simulink model "run_sim_paper_scenario"  (R2020a)
settings: Solver=ode4  StartTime=0.0  StopTime=30.0  FixedStep=0.01  RelTol=1e-3
values from neighbouring files (symbols this model uses):
  alfa_theta = 20    [init_sim_paper_scenario.m]
  alfa_theta_obs = 100    [init_sim_paper_scenario.m]
  beta1 = 1.2    [init_sim_paper_scenario.m]
  beta2 = 0.8    [init_sim_paper_scenario.m]
  beta_Phi_1 = pp0 * cal_frac_squ( 3, p_p0_plus_1, q_p0_plus_1 )                          * cal_frac_squ( eps_s_bar / pi, p_p0_min_2, q_p0_min_2 )                          / ( 2 * ( 2 * pp0 - 1 ) * tanh( gamma0 * ( eps_s_bar / pi ) / 2 ) )                          - ( cal_frac_squ( 3, p_p0_plus_1, q_p0_plus_1 ) * gamma0 / ( 4 * ( 2 * pp0 -1 ) ) )                          * cal_frac_squ( eps_s_bar / pi, p_p0_min_ ...(+136 chars)    [init_sim_paper_scenario.m]
  beta_Phi_2 = ( 1 - pp0 ) * cal_frac_squ( 3, p_p0_plus_1, q_p0_plus_1 )                          / ( 2 * ( 1 - 2 * pp0 ) * cal_frac_squ( eps_s_bar / pi, p_p0_0, q_p0_0 ) * tanh( gamma0 * ( eps_s_bar / pi ) / 2 ) )                          - ( cal_frac_squ( 3, p_p0_plus_1, q_p0_plus_1 ) * gamma0 / ( 4 * ( 1 - 2 * pp0 ) ) )                          * cal_frac_squ( eps_s_bar / pi, p_1_min_p0, q_1_min_p0 )          ...(+112 chars)    [init_sim_paper_scenario.m]
  c1_diff_sigma_bar_v = diag([25; 30; 20])    [init_sim_paper_scenario.m]
  c1_diff_sigma_bar_w = diag([12; 12; 12])    [init_sim_paper_scenario.m]
  c1_diff_ui = diag([25; 30; 20])    [init_sim_paper_scenario.m]
  c1v = diag([5.8; 6.5; 6.5])    [init_sim_paper_scenario.m]
  c2_diff_sigma_bar_v = diag([50; 50; 10])    [init_sim_paper_scenario.m]
  c2_diff_sigma_bar_w = diag([12; 12; 12])    [init_sim_paper_scenario.m]
  c2_diff_ui = diag([50; 50; 10])    [init_sim_paper_scenario.m]
  c2v = diag([5.8; 6.5; 6.5])    [init_sim_paper_scenario.m]
  c3_diff_sigma_bar_v = diag([15; 15; 10])    [init_sim_paper_scenario.m]
  c3_diff_sigma_bar_w = diag([15; 15; 15])    [init_sim_paper_scenario.m]
  c3_diff_ui = diag([15; 15; 10])    [init_sim_paper_scenario.m]
  c3v = diag([4.8; 6.4; 6.0])    [init_sim_paper_scenario.m]
  c_w_1 = diag( [20; 15; 15] )    [init_sim_paper_scenario.m]
  c_w_2 = diag( [20; 15; 15] )    [init_sim_paper_scenario.m]
  c_w_3 = diag( [2; 2; 2] )    [init_sim_paper_scenario.m]
  cS0 = diag( [4.5; 4.5; 4.5] )    [init_sim_paper_scenario.m]
  delta_p_i_0 = zeros(3, NF)    [init_sim_paper_scenario.m]
  delta_v_i_0 = zeros(3, NF)    [init_sim_paper_scenario.m]
  dp_aa_t = 0.2 * ones(3, 5) + ( 1.0 - 0.2 ) * rand(3, 5)    [init_sim_paper_scenario.m]
  dp_ff_t = [ 0.4 * ones(1, 5) + ( 1.0 - 0.4 ) * rand(1, 5);                      0.4 * ones(1, 5) + ( 1.0 - 0.4 ) * rand(1, 5);                      0.2 * ones(1, 5) + ( 0.6 - 0.2 ) * rand(1, 5) ]    [init_sim_paper_scenario.m]
  dp_phi_t = ( - pi / 2 ) * ones(3, 5) + ( pi / 2 - ( - pi / 2 ) ) * rand(3, 5)    [init_sim_paper_scenario.m]
  dw_aa_t = 0.2 * ones(3, 5) + ( 1.0 - 0.2 ) * rand(3, 5)    [init_sim_paper_scenario.m]
  dw_ff_t = [ 0.4 * ones(1, 5) + ( 1.0 - 0.4 ) * rand(1, 5);                      0.4 * ones(1, 5) + ( 1.0 - 0.4 ) * rand(1, 5);                      0.2 * ones(1, 5) + ( 0.6 - 0.2 ) * rand(1, 5) ]    [init_sim_paper_scenario.m]
  dw_phi_t = ( - pi / 2 ) * ones(3, 5) + ( pi / 2 - ( - pi / 2 ) ) * rand(3, 5)    [init_sim_paper_scenario.m]
  dwci_init = zeros(3,5)    [init_sim_paper_scenario.m]
  eps_s_bar_div_pi = eps_s_bar / pi    (= 0.03)    [init_sim_paper_scenario.m]
  etai_0 = zeros(3,5)    [init_sim_paper_scenario.m]
  gamma0 = 20    [init_sim_paper_scenario.m]
  h1w = diag([20.0; 20.0; 20.0])    [init_sim_paper_scenario.m]
  h2w = diag([30.0; 35.0; 35.0])    [init_sim_paper_scenario.m]
  h3w = diag([30.0; 25.0; 30.0])    [init_sim_paper_scenario.m]
  Ji = zeros(3,3,NF)    [init_sim_paper_scenario.m]
  k_J_0 = diag( [1; 1; 1] )    [init_sim_paper_scenario.m]
  kai_1_t = 0.02    [init_sim_paper_scenario.m]
  kai_3_t = 0.1    [init_sim_paper_scenario.m]
  kai_chi_1 = diag([6; 6; 6])    [init_sim_paper_scenario.m]
  kai_chi_2 = diag([6; 6; 6])    [init_sim_paper_scenario.m]
  kai_u_1 = diag([8; 8; 8])    [init_sim_paper_scenario.m]
  kai_u_2 = diag([8; 8; 8])    [init_sim_paper_scenario.m]
  ksii_0 = zeros(3,5)    [init_sim_paper_scenario.m]
  l1v = diag([20; 20; 20])    [init_sim_paper_scenario.m]
  l2v = diag([30; 30; 30])    [init_sim_paper_scenario.m]
  Lamd_diff_sigma_bar_v = 0.5    [init_sim_paper_scenario.m]
  Lamd_diff_sigma_bar_w = 0.8    [init_sim_paper_scenario.m]
  Lamd_diff_ui = 0.8    [init_sim_paper_scenario.m]
  mass_i = zeros(1,NF)    [init_sim_paper_scenario.m]
  Mii = diag([1;0;0;0;1])    [init_sim_paper_scenario.m]
  mu_c_theta = 100    [init_sim_paper_scenario.m]
  mu_d_w = 100    [init_sim_paper_scenario.m]
  pos0 = zeros(3, 1)    [init_sim_paper_scenario.m]
  pp0 = 8 / 11    (= 0.727272727273)    [init_sim_paper_scenario.m]    (also in plot_sim_paper_scenario.m = plot3( ksi0(1, kkt), ksi0(2, kkt), ksi0(3, kkt),            )
  PZ0 = P0(3)    [init_sim_paper_scenario.m]
  PZ1 = 10    [init_sim_paper_scenario.m]
  Qci_init = repmat([1;0;0;0],1,NF)    [init_sim_paper_scenario.m]
  R0 = 4    [init_sim_paper_scenario.m]
  R1 = 8    [init_sim_paper_scenario.m]
  Rci_init = zeros(3,3,NF)    [init_sim_paper_scenario.m]
  Ri_init = zeros(3,3,NF)    [init_sim_paper_scenario.m]
  Rx2 = 10    [init_sim_paper_scenario.m]
  Ry2 = 6    [init_sim_paper_scenario.m]
  Rz2 = 4    [init_sim_paper_scenario.m]
  T0 = 0    [init_sim_paper_scenario.m]
  T1 = tseq1    (= 10)    [init_sim_paper_scenario.m]
  T12 = tseq1 + tseq12    (= 20)    [init_sim_paper_scenario.m]
  T2 = tseq1 + tseq12 + tseq2    (= 30)    [init_sim_paper_scenario.m]
  theta0 = ( 2 / 5 ) * pi    (= 1.25663706144)    [init_sim_paper_scenario.m]
  thr_p_plus_1 = cal_frac_squ( 3, p_p0_plus_1, q_p0_plus_1 )    [init_sim_paper_scenario.m]
  ui_init = zeros(3,NF)    [init_sim_paper_scenario.m]
  vel0 = zeros(3, 1)    [init_sim_paper_scenario.m]
  wci_init = zeros(3,5)    [init_sim_paper_scenario.m]
  Wij = [0,0,1,0,0;              0,0,1,1,0;              1,0,0,0,1;              0,1,1,0,0;              0,0,1,0,0]    [init_sim_paper_scenario.m]
  X1 = 8    [init_sim_paper_scenario.m]
  X2 = 2    [init_sim_paper_scenario.m]
  X3 = 3    [init_sim_paper_scenario.m]
  Y1 = 10    [init_sim_paper_scenario.m]
  Y2 = 2    [init_sim_paper_scenario.m]
  Y3 = 4    [init_sim_paper_scenario.m]
  Z1 = 4    [init_sim_paper_scenario.m]
  Z2 = -6    [init_sim_paper_scenario.m]
  Z3 = 2    [init_sim_paper_scenario.m]
  zeta_diff_sigma_bar_v = 0.08    [init_sim_paper_scenario.m]
  zeta_diff_sigma_bar_w = 0.3    [init_sim_paper_scenario.m]
  zeta_diff_ui = 0.05    [init_sim_paper_scenario.m]
undefined symbols (not defined in the file or in its folder): cal_frac_squ, p_2_p0, p_alfav1, p_alfav2, p_alfaw1, p_alfaw2, p_beta1, p_beta2, p_beta_w_1, p_beta_w_2, p_dbeta1, p_dbeta2, p_gamma1_pos, p_gamma1_vel, p_gamma2_pos, p_gamma2_vel, p_p0_min_1, p_p0_plus_1, q_2_p0, q_alfav1, q_alfav2, q_alfaw1, q_alfaw2, q_beta1, q_beta2, q_beta_w_1, q_beta_w_2, q_dbeta1, q_dbeta2, q_gamma1_pos, q_gamma1_vel, q_gamma2_pos, q_gamma2_vel, q_p0_min_1, q_p0_plus_1, Qei_init, Qi_init, Rei_init, V_Phi_Rei_init, wei_init, wi_init
(part 7 of 10)

== matlab function run_sim_paper_scenario/Qi dynam agent 4 ==
  data: Qi_vec input; dQi_4 output; wi_vec input
function dQi_4 = fcn(Qi_vec, wi_vec)
%%%% update quaternion dynamics
iiuav = 4;

wi = wi_vec(:,iiuav);
thetai = Qi_vec(1,iiuav);
qi = Qi_vec(2:4,iiuav);

GammaQi = zeros(4,3);
GammaQi(1,:) = -(qi');
GammaQi(2:4,:) = thetai*eye(3,3) + cal_askew_mat(qi);
dQi_4 = (1/2)*GammaQi*wi;

end

== matlab function run_sim_paper_scenario/Qi dynam agent 5 ==
  data: Qi_vec input; dQi_5 output; wi_vec input
function dQi_5 = fcn(Qi_vec, wi_vec)
%%%% update quaternion dynamics
iiuav = 5;

wi = wi_vec(:,iiuav);
thetai = Qi_vec(1,iiuav);
qi = Qi_vec(2:4,iiuav);

GammaQi = zeros(4,3);
GammaQi(1,:) = -(qi');
GammaQi(2:4,:) = thetai*eye(3,3) + cal_askew_mat(qi);
dQi_5 = (1/2)*GammaQi*wi;

end

== matlab function run_sim_paper_scenario/trans to column5 ==
  data: x input; y output
function y = fcn(x)
y = x(:);

== matlab function run_sim_paper_scenario/cal Fi_S agent 1 ==
  data: cS0 input; Ji input; wi_vec input; wci_vec input; wei_vec input; Fi_S_1 output; dwci_vec input; Rei_vec input; Phi_bar_psi_e_vec input
function Fi_S_1 = fcn(cS0, Ji, wi_vec, wci_vec, wei_vec, dwci_vec, Rei_vec, Phi_bar_psi_e_vec)
%%%% compensation term
iiuav = 1;
Fi_S_1 = -cal_askew_mat( wi_vec(:,iiuav) ) * Ji(:,:,iiuav) * wi_vec(:,iiuav) ...
                + Ji(:,:,iiuav) * cal_askew_mat( wei_vec(:,iiuav) ) * ( Rei_vec(:,:,iiuav)' ) * wci_vec(:,iiuav) ...
                - Ji(:,:,iiuav) * ( Rei_vec(:,:,iiuav)' ) * dwci_vec(:,iiuav) ...
                + cS0 * Ji(:,:,iiuav) * Phi_bar_psi_e_vec(:,iiuav);

== matlab function run_sim_paper_scenario/cal Fi_S agent 2 ==
  data: cS0 input; Ji input; wi_vec input; wci_vec input; wei_vec input; Fi_S_2 output; dwci_vec input; Rei_vec input; Phi_bar_psi_e_vec input
function Fi_S_2 = fcn(cS0, Ji, wi_vec, wci_vec, wei_vec, dwci_vec, Rei_vec, Phi_bar_psi_e_vec)
%%%% compensation term
iiuav = 2;
Fi_S_2 = -cal_askew_mat( wi_vec(:,iiuav) ) * Ji(:,:,iiuav) * wi_vec(:,iiuav) ...
                + Ji(:,:,iiuav) * cal_askew_mat( wei_vec(:,iiuav) ) * ( Rei_vec(:,:,iiuav)' ) * wci_vec(:,iiuav) ...
                - Ji(:,:,iiuav) * ( Rei_vec(:,:,iiuav)' ) * dwci_vec(:,iiuav) ...
                + cS0 * Ji(:,:,iiuav) * Phi_bar_psi_e_vec(:,iiuav);

== matlab function run_sim_paper_scenario/cal Fi_S agent 3 ==
  data: cS0 input; Ji input; wi_vec input; wci_vec input; wei_vec input; Fi_S_3 output; dwci_vec input; Rei_vec input; Phi_bar_psi_e_vec input
function Fi_S_3 = fcn(cS0, Ji, wi_vec, wci_vec, wei_vec, dwci_vec, Rei_vec, Phi_bar_psi_e_vec)
%%%% compensation term
iiuav = 3;
Fi_S_3 = -cal_askew_mat( wi_vec(:,iiuav) ) * Ji(:,:,iiuav) * wi_vec(:,iiuav) ...
                + Ji(:,:,iiuav) * cal_askew_mat( wei_vec(:,iiuav) ) * ( Rei_vec(:,:,iiuav)' ) * wci_vec(:,iiuav) ...
                - Ji(:,:,iiuav) * ( Rei_vec(:,:,iiuav)' ) * dwci_vec(:,iiuav) ...
                + cS0 * Ji(:,:,iiuav) * Phi_bar_psi_e_vec(:,iiuav);

== matlab function run_sim_paper_scenario/cal Fi_S agent 4 ==
  data: cS0 input; Ji input; wi_vec input; wci_vec input; wei_vec input; Fi_S_4 output; dwci_vec input; Rei_vec input; Phi_bar_psi_e_vec input
function Fi_S_4 = fcn(cS0, Ji, wi_vec, wci_vec, wei_vec, dwci_vec, Rei_vec, Phi_bar_psi_e_vec)
%%%% compensation term
iiuav = 4;
Fi_S_4 = -cal_askew_mat( wi_vec(:,iiuav) ) * Ji(:,:,iiuav) * wi_vec(:,iiuav) ...
                + Ji(:,:,iiuav) * cal_askew_mat( wei_vec(:,iiuav) ) * ( Rei_vec(:,:,iiuav)' ) * wci_vec(:,iiuav) ...
                - Ji(:,:,iiuav) * ( Rei_vec(:,:,iiuav)' ) * dwci_vec(:,iiuav) ...
                + cS0 * Ji(:,:,iiuav) * Phi_bar_psi_e_vec(:,iiuav);

== matlab function run_sim_paper_scenario/cal Fi_S agent 5 ==
  data: cS0 input; Ji input; wi_vec input; wci_vec input; wei_vec input; Fi_S_5 output; dwci_vec input; Rei_vec input; Phi_bar_psi_e_vec input
function Fi_S_5 = fcn(cS0, Ji, wi_vec, wci_vec, wei_vec, dwci_vec, Rei_vec, Phi_bar_psi_e_vec)
%%%% compensation term
iiuav = 5;
Fi_S_5 = -cal_askew_mat( wi_vec(:,iiuav) ) * Ji(:,:,iiuav) * wi_vec(:,iiuav) ...
                + Ji(:,:,iiuav) * cal_askew_mat( wei_vec(:,iiuav) ) * ( Rei_vec(:,:,iiuav)' ) * wci_vec(:,iiuav) ...
                - Ji(:,:,iiuav) * ( Rei_vec(:,:,iiuav)' ) * dwci_vec(:,iiuav) ...
                + cS0 * Ji(:,:,iiuav) * Phi_bar_psi_e_vec(:,iiuav);

== matlab function run_sim_paper_scenario/cal abs 7 ==
  data: x input; y output
function y = fcn(x)
y = abs(x(:));

== matlab function run_sim_paper_scenario/cal Phi_bar_psi_e agent 1 ==
  data: pp0 input; Phi_bar_psi_e_node_1 output; beta_Phi_1 input; beta_Phi_2 input; thr_p_plus_1 input; gamma0 input; eps_s_bar_div_pi input; wei_vec input; S_bar_vec input; V_Phi_Rei_div_pi_vec input; V_Phi_Rei_squ_p_min_1_vec input; V_Phi_Rei_squ_p_plus_1_vec input; V_Phi_Rei_squ_2p_vec input
function Phi_bar_psi_e_node_1 = fcn(pp0, beta_Phi_1, beta_Phi_2, thr_p_plus_1, gamma0, ...
                                                                    eps_s_bar_div_pi, wei_vec, S_bar_vec, V_Phi_Rei_div_pi_vec, ...
                                                                    V_Phi_Rei_squ_p_min_1_vec, V_Phi_Rei_squ_p_plus_1_vec, V_Phi_Rei_squ_2p_vec)
%%%% intermediate auxiliary switching rotational error
iiuav = 1;
Phi_bar_psi_e_node_1 = zeros(3,1);
for kk = 1:3
    if S_bar_vec(kk, iiuav) == 0
        Phi_bar_psi_e_node_1(kk, 1) = thr_p_plus_1 * ( pp0 + 1 ) * V_Phi_Rei_div_pi_vec(kk, iiuav) ...
                                                                * V_Phi_Rei_squ_p_min_1_vec(kk, iiuav) * wei_vec(kk, iiuav) ...
                                                                / ( 2 * tanh( ( gamma0 / 2 ) * V_Phi_Rei_div_pi_vec(kk, iiuav) ) ) ...
                                                                + ( thr_p_plus_1 * gamma0 / 4 ) * V_Phi_Rei_squ_p_plus_1_vec(kk, iiuav) ...
                                                                * ( ( sech( ( gamma0 / 2 ) * V_Phi_Rei_div_pi_vec(kk, iiuav) ) ...
                                                                / tanh( ( gamma0 / 2 ) * V_Phi_Rei_div_pi_vec(kk, iiuav) ) ) ^ 2 ) * wei_vec(kk, iiuav);
    else
        if abs( V_Phi_Rei_div_pi_vec ) > eps_s_bar_div_pi
            Phi_bar_psi_e_node_1(kk, 1) = thr_p_plus_1 * ( pp0 + 1 ) * V_Phi_Rei_div_pi_vec(kk, iiuav) ...
                                                                    * V_Phi_Rei_squ_p_min_1_vec(kk, iiuav) * wei_vec(kk, iiuav) ...
                                                                    / ( 2 * tanh( ( gamma0 / 2 ) * V_Phi_Rei_div_pi_vec(kk, iiuav) ) ) ...
                                                                    + ( thr_p_plus_1 * gamma0 / 4 ) * V_Phi_Rei_squ_p_plus_1_vec(kk, iiuav) ...
                                                                    * ( ( sech( ( gamma0 / 2 ) * V_Phi_Rei_div_pi_vec(kk, iiuav) ) ...
                                                                    / tanh( ( gamma0 / 2 ) * V_Phi_Rei_div_pi_vec(kk, iiuav) ) ) ^ 2 ) * wei_vec(kk, iiuav);
        else
            Phi_bar_psi_e_node_1(kk, 1) = 2 * beta_Phi_1 * ( ( abs( V_Phi_Rei_div_pi_vec(kk, iiuav) ) ) ^ 2 ) * wei_vec(kk, iiuav) ...
                                                                    + ( 2 * pp0 + 1 ) * beta_Phi_2 * V_Phi_Rei_squ_2p_vec(kk, iiuav) * wei_vec(kk, iiuav);
        end
    end
end

== matlab function run_sim_paper_scenario/cal Phi_bar_psi_e agent 2 ==
  data: pp0 input; Phi_bar_psi_e_node_2 output; beta_Phi_1 input; beta_Phi_2 input; thr_p_plus_1 input; gamma0 input; eps_s_bar_div_pi input; wei_vec input; S_bar_vec input; V_Phi_Rei_div_pi_vec input; V_Phi_Rei_squ_p_min_1_vec input; V_Phi_Rei_squ_p_plus_1_vec input; V_Phi_Rei_squ_2p_vec input
function Phi_bar_psi_e_node_2 = fcn(pp0, beta_Phi_1, beta_Phi_2, thr_p_plus_1, gamma0, ...
                                                                    eps_s_bar_div_pi, wei_vec, S_bar_vec, V_Phi_Rei_div_pi_vec, ...
                                                                    V_Phi_Rei_squ_p_min_1_vec, V_Phi_Rei_squ_p_plus_1_vec, V_Phi_Rei_squ_2p_vec)
%%%% intermediate auxiliary switching rotational error
iiuav = 2;
Phi_bar_psi_e_node_2 = zeros(3,1);
for kk = 1:3
    if S_bar_vec(kk, iiuav) == 0
        Phi_bar_psi_e_node_2(kk, 1) = thr_p_plus_1 * ( pp0 + 1 ) * V_Phi_Rei_div_pi_vec(kk, iiuav) ...
                                                                * V_Phi_Rei_squ_p_min_1_vec(kk, iiuav) * wei_vec(kk, iiuav) ...
                                                                / ( 2 * tanh( ( gamma0 / 2 ) * V_Phi_Rei_div_pi_vec(kk, iiuav) ) ) ...
                                                                + ( thr_p_plus_1 * gamma0 / 4 ) * V_Phi_Rei_squ_p_plus_1_vec(kk, iiuav) ...
                                                                * ( ( sech( ( gamma0 / 2 ) * V_Phi_Rei_div_pi_vec(kk, iiuav) ) ...
                                                                / tanh( ( gamma0 / 2 ) * V_Phi_Rei_div_pi_vec(kk, iiuav) ) ) ^ 2 ) * wei_vec(kk, iiuav);
    else
        if abs( V_Phi_Rei_div_pi_vec ) > eps_s_bar_div_pi
            Phi_bar_psi_e_node_2(kk, 1) = thr_p_plus_1 * ( pp0 + 1 ) * V_Phi_Rei_div_pi_vec(kk, iiuav) ...
                                                                    * V_Phi_Rei_squ_p_min_1_vec(kk, iiuav) * wei_vec(kk, iiuav) ...
                                                                    / ( 2 * tanh( ( gamma0 / 2 ) * V_Phi_Rei_div_pi_vec(kk, iiuav) ) ) ...
                                                                    + ( thr_p_plus_1 * gamma0 / 4 ) * V_Phi_Rei_squ_p_plus_1_vec(kk, iiuav) ...
                                                                    * ( ( sech( ( gamma0 / 2 ) * V_Phi_Rei_div_pi_vec(kk, iiuav) ) ...
                                                                    / tanh( ( gamma0 / 2 ) * V_Phi_Rei_div_pi_vec(kk, iiuav) ) ) ^ 2 ) * wei_vec(kk, iiuav);
        else
            Phi_bar_psi_e_node_2(kk, 1) = 2 * beta_Phi_1 * ( ( abs( V_Phi_Rei_div_pi_vec(kk, iiuav) ) ) ^ 2 ) * wei_vec(kk, iiuav) ...
                                                                    + ( 2 * pp0 + 1 ) * beta_Phi_2 * V_Phi_Rei_squ_2p_vec(kk, iiuav) * wei_vec(kk, iiuav);
        end
    end
end

== matlab function run_sim_paper_scenario/cal Phi_bar_psi_e agent 3 ==
  data: pp0 input; Phi_bar_psi_e_node_3 output; beta_Phi_1 input; beta_Phi_2 input; thr_p_plus_1 input; gamma0 input; eps_s_bar_div_pi input; wei_vec input; S_bar_vec input; V_Phi_Rei_div_pi_vec input; V_Phi_Rei_squ_p_min_1_vec input; V_Phi_Rei_squ_p_plus_1_vec input; V_Phi_Rei_squ_2p_vec input
function Phi_bar_psi_e_node_3 = fcn(pp0, beta_Phi_1, beta_Phi_2, thr_p_plus_1, gamma0, ...
                                                                    eps_s_bar_div_pi, wei_vec, S_bar_vec, V_Phi_Rei_div_pi_vec, ...
                                                                    V_Phi_Rei_squ_p_min_1_vec, V_Phi_Rei_squ_p_plus_1_vec, V_Phi_Rei_squ_2p_vec)
%%%% intermediate auxiliary switching rotational error
iiuav = 3;
Phi_bar_psi_e_node_3 = zeros(3,1);
for kk = 1:3
    if S_bar_vec(kk, iiuav) == 0
        Phi_bar_psi_e_node_3(kk, 1) = thr_p_plus_1 * ( pp0 + 1 ) * V_Phi_Rei_div_pi_vec(kk, iiuav) ...
                                                                * V_Phi_Rei_squ_p_min_1_vec(kk, iiuav) * wei_vec(kk, iiuav) ...
                                                                / ( 2 * tanh( ( gamma0 / 2 ) * V_Phi_Rei_div_pi_vec(kk, iiuav) ) ) ...
                                                                + ( thr_p_plus_1 * gamma0 / 4 ) * V_Phi_Rei_squ_p_plus_1_vec(kk, iiuav) ...
                                                                * ( ( sech( ( gamma0 / 2 ) * V_Phi_Rei_div_pi_vec(kk, iiuav) ) ...
                                                                / tanh( ( gamma0 / 2 ) * V_Phi_Rei_div_pi_vec(kk, iiuav) ) ) ^ 2 ) * wei_vec(kk, iiuav);
    else
        if abs( V_Phi_Rei_div_pi_vec ) > eps_s_bar_div_pi
            Phi_bar_psi_e_node_3(kk, 1) = thr_p_plus_1 * ( pp0 + 1 ) * V_Phi_Rei_div_pi_vec(kk, iiuav) ...
                                                                    * V_Phi_Rei_squ_p_min_1_vec(kk, iiuav) * wei_vec(kk, iiuav) ...
                                                                    / ( 2 * tanh( ( gamma0 / 2 ) * V_Phi_Rei_div_pi_vec(kk, iiuav) ) ) ...
                                                                    + ( thr_p_plus_1 * gamma0 / 4 ) * V_Phi_Rei_squ_p_plus_1_vec(kk, iiuav) ...
                                                                    * ( ( sech( ( gamma0 / 2 ) * V_Phi_Rei_div_pi_vec(kk, iiuav) ) ...
                                                                    / tanh( ( gamma0 / 2 ) * V_Phi_Rei_div_pi_vec(kk, iiuav) ) ) ^ 2 ) * wei_vec(kk, iiuav);
        else
            Phi_bar_psi_e_node_3(kk, 1) = 2 * beta_Phi_1 * ( ( abs( V_Phi_Rei_div_pi_vec(kk, iiuav) ) ) ^ 2 ) * wei_vec(kk, iiuav) ...
                                                                    + ( 2 * pp0 + 1 ) * beta_Phi_2 * V_Phi_Rei_squ_2p_vec(kk, iiuav) * wei_vec(kk, iiuav);
        end
    end
end

== matlab function run_sim_paper_scenario/cal Phi_bar_psi_e agent 4 ==
  data: pp0 input; Phi_bar_psi_e_node_4 output; beta_Phi_1 input; beta_Phi_2 input; thr_p_plus_1 input; gamma0 input; eps_s_bar_div_pi input; wei_vec input; S_bar_vec input; V_Phi_Rei_div_pi_vec input; V_Phi_Rei_squ_p_min_1_vec input; V_Phi_Rei_squ_p_plus_1_vec input; V_Phi_Rei_squ_2p_vec input
function Phi_bar_psi_e_node_4 = fcn(pp0, beta_Phi_1, beta_Phi_2, thr_p_plus_1, gamma0, ...
                                                                    eps_s_bar_div_pi, wei_vec, S_bar_vec, V_Phi_Rei_div_pi_vec, ...
                                                                    V_Phi_Rei_squ_p_min_1_vec, V_Phi_Rei_squ_p_plus_1_vec, V_Phi_Rei_squ_2p_vec)
%%%% intermediate auxiliary switching rotational error
iiuav = 4;
Phi_bar_psi_e_node_4 = zeros(3,1);
for kk = 1:3
    if S_bar_vec(kk, iiuav) == 0
        Phi_bar_psi_e_node_4(kk, 1) = thr_p_plus_1 * ( pp0 + 1 ) * V_Phi_Rei_div_pi_vec(kk, iiuav) ...
                                                                * V_Phi_Rei_squ_p_min_1_vec(kk, iiuav) * wei_vec(kk, iiuav) ...
                                                                / ( 2 * tanh( ( gamma0 / 2 ) * V_Phi_Rei_div_pi_vec(kk, iiuav) ) ) ...
                                                                + ( thr_p_plus_1 * gamma0 / 4 ) * V_Phi_Rei_squ_p_plus_1_vec(kk, iiuav) ...
                                                                * ( ( sech( ( gamma0 / 2 ) * V_Phi_Rei_div_pi_vec(kk, iiuav) ) ...
                                                                / tanh( ( gamma0 / 2 ) * V_Phi_Rei_div_pi_vec(kk, iiuav) ) ) ^ 2 ) * wei_vec(kk, iiuav);
    else
        if abs( V_Phi_Rei_div_pi_vec ) > eps_s_bar_div_pi
            Phi_bar_psi_e_node_4(kk, 1) = thr_p_plus_1 * ( pp0 + 1 ) * V_Phi_Rei_div_pi_vec(kk, iiuav) ...
                                                                    * V_Phi_Rei_squ_p_min_1_vec(kk, iiuav) * wei_vec(kk, iiuav) ...
                                                                    / ( 2 * tanh( ( gamma0 / 2 ) * V_Phi_Rei_div_pi_vec(kk, iiuav) ) ) ...
                                                                    + ( thr_p_plus_1 * gamma0 / 4 ) * V_Phi_Rei_squ_p_plus_1_vec(kk, iiuav) ...
                                                                    * ( ( sech( ( gamma0 / 2 ) * V_Phi_Rei_div_pi_vec(kk, iiuav) ) ...
                                                                    / tanh( ( gamma0 / 2 ) * V_Phi_Rei_div_pi_vec(kk, iiuav) ) ) ^ 2 ) * wei_vec(kk, iiuav);
        else
            Phi_bar_psi_e_node_4(kk, 1) = 2 * beta_Phi_1 * ( ( abs( V_Phi_Rei_div_pi_vec(kk, iiuav) ) ) ^ 2 ) * wei_vec(kk, iiuav) ...
                                                                    + ( 2 * pp0 + 1 ) * beta_Phi_2 * V_Phi_Rei_squ_2p_vec(kk, iiuav) * wei_vec(kk, iiuav);
        end
    end
end

== matlab function run_sim_paper_scenario/cal abs 8 ==
  data: x input; y output
function y = fcn(x)
y = abs(x(:));

== matlab function run_sim_paper_scenario/cal Phi_bar_psi_e agent 5 ==
  data: pp0 input; Phi_bar_psi_e_node_5 output; beta_Phi_1 input; beta_Phi_2 input; thr_p_plus_1 input; gamma0 input; eps_s_bar_div_pi input; wei_vec input; S_bar_vec input; V_Phi_Rei_div_pi_vec input; V_Phi_Rei_squ_p_min_1_vec input; V_Phi_Rei_squ_p_plus_1_vec input; V_Phi_Rei_squ_2p_vec input
function Phi_bar_psi_e_node_5 = fcn(pp0, beta_Phi_1, beta_Phi_2, thr_p_plus_1, gamma0, ...
                                                                    eps_s_bar_div_pi, wei_vec, S_bar_vec, V_Phi_Rei_div_pi_vec, ...
                                                                    V_Phi_Rei_squ_p_min_1_vec, V_Phi_Rei_squ_p_plus_1_vec, V_Phi_Rei_squ_2p_vec)
%%%% intermediate auxiliary switching rotational error
iiuav = 5;
Phi_bar_psi_e_node_5 = zeros(3,1);
for kk = 1:3
    if S_bar_vec(kk, iiuav) == 0
        Phi_bar_psi_e_node_5(kk, 1) = thr_p_plus_1 * ( pp0 + 1 ) * V_Phi_Rei_div_pi_vec(kk, iiuav) ...
                                                                * V_Phi_Rei_squ_p_min_1_vec(kk, iiuav) * wei_vec(kk, iiuav) ...
                                                                / ( 2 * tanh( ( gamma0 / 2 ) * V_Phi_Rei_div_pi_vec(kk, iiuav) ) ) ...
                                                                + ( thr_p_plus_1 * gamma0 / 4 ) * V_Phi_Rei_squ_p_plus_1_vec(kk, iiuav) ...
                                                                * ( ( sech( ( gamma0 / 2 ) * V_Phi_Rei_div_pi_vec(kk, iiuav) ) ...
                                                                / tanh( ( gamma0 / 2 ) * V_Phi_Rei_div_pi_vec(kk, iiuav) ) ) ^ 2 ) * wei_vec(kk, iiuav);
    else
        if abs( V_Phi_Rei_div_pi_vec ) > eps_s_bar_div_pi
            Phi_bar_psi_e_node_5(kk, 1) = thr_p_plus_1 * ( pp0 + 1 ) * V_Phi_Rei_div_pi_vec(kk, iiuav) ...
                                                                    * V_Phi_Rei_squ_p_min_1_vec(kk, iiuav) * wei_vec(kk, iiuav) ...
                                                                    / ( 2 * tanh( ( gamma0 / 2 ) * V_Phi_Rei_div_pi_vec(kk, iiuav) ) ) ...
                                                                    + ( thr_p_plus_1 * gamma0 / 4 ) * V_Phi_Rei_squ_p_plus_1_vec(kk, iiuav) ...
                                                                    * ( ( sech( ( gamma0 / 2 ) * V_Phi_Rei_div_pi_vec(kk, iiuav) ) ...
                                                                    / tanh( ( gamma0 / 2 ) * V_Phi_Rei_div_pi_vec(kk, iiuav) ) ) ^ 2 ) * wei_vec(kk, iiuav);
        else
            Phi_bar_psi_e_node_5(kk, 1) = 2 * beta_Phi_1 * ( ( abs( V_Phi_Rei_div_pi_vec(kk, iiuav) ) ) ^ 2 ) * wei_vec(kk, iiuav) ...
                                                                    + ( 2 * pp0 + 1 ) * beta_Phi_2 * V_Phi_Rei_squ_2p_vec(kk, iiuav) * wei_vec(kk, iiuav);
        end
    end
end

== matlab function run_sim_paper_scenario/cal Phi_psi_e agent 1 ==
  data: Phi_psi_e_node_1 output; beta_Phi_1 input; beta_Phi_2 input; gamma0 input; thr_p_plus_1 input; eps_s_bar_div_pi input; S_bar_vec input; V_Phi_Rei_div_pi_vec input; V_Phi_Rei_squ_p_plus_1_vec input; V_Phi_Rei_squ_2p_vec input
function Phi_psi_e_node_1 = fcn(beta_Phi_1, beta_Phi_2, gamma0, thr_p_plus_1, eps_s_bar_div_pi, ...
                                                            S_bar_vec, V_Phi_Rei_div_pi_vec, ...
                                                            V_Phi_Rei_squ_p_plus_1_vec, V_Phi_Rei_squ_2p_vec)
%%%% intermediate switching rotational error
iiuav = 1;
Phi_psi_e_node_1 = zeros(3,1);
for kk = 1:3
    if S_bar_vec(kk, iiuav) == 0
        Phi_psi_e_node_1(kk, 1) = ( thr_p_plus_1 * pi * V_Phi_Rei_squ_p_plus_1_vec(kk,iiuav) ) ...
                                                        / ( 2 * tanh( ( gamma0 / 2 ) * V_Phi_Rei_div_pi_vec(kk,iiuav) ) );
    else
        if abs( V_Phi_Rei_div_pi_vec ) > eps_s_bar_div_pi
            Phi_psi_e_node_1(kk, 1) = ( thr_p_plus_1 * pi * V_Phi_Rei_squ_p_plus_1_vec(kk,iiuav) ) ...
                                                            / ( 2 * tanh( ( gamma0 / 2 ) * V_Phi_Rei_div_pi_vec(kk,iiuav) ) );
        else
            Phi_psi_e_node_1(kk, 1) = V_Phi_Rei_div_pi_vec(kk, iiuav) * pi * ...
                                                            ( beta_Phi_1 * ( abs( V_Phi_Rei_div_pi_vec(kk, iiuav) ) ^ 2 ) ...
                                                            + beta_Phi_2 * V_Phi_Rei_squ_2p_vec(kk, iiuav) );
        end
    end
end

== matlab function run_sim_paper_scenario/cal Phi_psi_e agent 2 ==
  data: Phi_psi_e_node_2 output; beta_Phi_1 input; beta_Phi_2 input; gamma0 input; thr_p_plus_1 input; eps_s_bar_div_pi input; S_bar_vec input; V_Phi_Rei_div_pi_vec input; V_Phi_Rei_squ_p_plus_1_vec input; V_Phi_Rei_squ_2p_vec input
function Phi_psi_e_node_2 = fcn(beta_Phi_1, beta_Phi_2, gamma0, thr_p_plus_1, eps_s_bar_div_pi, ...
                                                            S_bar_vec, V_Phi_Rei_div_pi_vec, ...
                                                            V_Phi_Rei_squ_p_plus_1_vec, V_Phi_Rei_squ_2p_vec)
%%%% intermediate switching rotational error
iiuav = 2;
Phi_psi_e_node_2 = zeros(3,1);
for kk = 1:3
    if S_bar_vec(kk, iiuav) == 0
        Phi_psi_e_node_2(kk, 1) = ( thr_p_plus_1 * pi * V_Phi_Rei_squ_p_plus_1_vec(kk,iiuav) ) ...
                                                        / ( 2 * tanh( ( gamma0 / 2 ) * V_Phi_Rei_div_pi_vec(kk,iiuav) ) );
    else
        if abs( V_Phi_Rei_div_pi_vec ) > eps_s_bar_div_pi
            Phi_psi_e_node_2(kk, 1) = ( thr_p_plus_1 * pi * V_Phi_Rei_squ_p_plus_1_vec(kk,iiuav) ) ...
                                                            / ( 2 * tanh( ( gamma0 / 2 ) * V_Phi_Rei_div_pi_vec(kk,iiuav) ) );
        else
            Phi_psi_e_node_2(kk, 1) = V_Phi_Rei_div_pi_vec(kk, iiuav) * pi * ...
                                                            ( beta_Phi_1 * ( abs( V_Phi_Rei_div_pi_vec(kk, iiuav) ) ^ 2 ) ...
                                                            + beta_Phi_2 * V_Phi_Rei_squ_2p_vec(kk, iiuav) );
        end
    end
end

== matlab function run_sim_paper_scenario/cal Phi_psi_e agent 3 ==
  data: Phi_psi_e_node_3 output; beta_Phi_1 input; beta_Phi_2 input; gamma0 input; thr_p_plus_1 input; eps_s_bar_div_pi input; S_bar_vec input; V_Phi_Rei_div_pi_vec input; V_Phi_Rei_squ_p_plus_1_vec input; V_Phi_Rei_squ_2p_vec input
function Phi_psi_e_node_3 = fcn(beta_Phi_1, beta_Phi_2, gamma0, thr_p_plus_1, eps_s_bar_div_pi, ...
                                                            S_bar_vec, V_Phi_Rei_div_pi_vec, ...
                                                            V_Phi_Rei_squ_p_plus_1_vec, V_Phi_Rei_squ_2p_vec)
%%%% intermediate switching rotational error
iiuav = 3;
Phi_psi_e_node_3 = zeros(3,1);
for kk = 1:3
    if S_bar_vec(kk, iiuav) == 0
        Phi_psi_e_node_3(kk, 1) = ( thr_p_plus_1 * pi * V_Phi_Rei_squ_p_plus_1_vec(kk,iiuav) ) ...
                                                        / ( 2 * tanh( ( gamma0 / 2 ) * V_Phi_Rei_div_pi_vec(kk,iiuav) ) );
    else
        if abs( V_Phi_Rei_div_pi_vec ) > eps_s_bar_div_pi
            Phi_psi_e_node_3(kk, 1) = ( thr_p_plus_1 * pi * V_Phi_Rei_squ_p_plus_1_vec(kk,iiuav) ) ...
                                                            / ( 2 * tanh( ( gamma0 / 2 ) * V_Phi_Rei_div_pi_vec(kk,iiuav) ) );
        else
            Phi_psi_e_node_3(kk, 1) = V_Phi_Rei_div_pi_vec(kk, iiuav) * pi * ...
                                                            ( beta_Phi_1 * ( abs( V_Phi_Rei_div_pi_vec(kk, iiuav) ) ^ 2 ) ...
                                                            + beta_Phi_2 * V_Phi_Rei_squ_2p_vec(kk, iiuav) );
        end
    end
end

== matlab function run_sim_paper_scenario/cal Phi_psi_e agent 4 ==
  data: Phi_psi_e_node_4 output; beta_Phi_1 input; beta_Phi_2 input; gamma0 input; thr_p_plus_1 input; eps_s_bar_div_pi input; S_bar_vec input; V_Phi_Rei_div_pi_vec input; V_Phi_Rei_squ_p_plus_1_vec input; V_Phi_Rei_squ_2p_vec input
function Phi_psi_e_node_4 = fcn(beta_Phi_1, beta_Phi_2, gamma0, thr_p_plus_1, eps_s_bar_div_pi, ...
                                                            S_bar_vec, V_Phi_Rei_div_pi_vec, ...
                                                            V_Phi_Rei_squ_p_plus_1_vec, V_Phi_Rei_squ_2p_vec)
%%%% intermediate switching rotational error
iiuav = 4;
Phi_psi_e_node_4 = zeros(3,1);
for kk = 1:3
    if S_bar_vec(kk, iiuav) == 0
        Phi_psi_e_node_4(kk, 1) = ( thr_p_plus_1 * pi * V_Phi_Rei_squ_p_plus_1_vec(kk,iiuav) ) ...
                                                        / ( 2 * tanh( ( gamma0 / 2 ) * V_Phi_Rei_div_pi_vec(kk,iiuav) ) );
    else
        if abs( V_Phi_Rei_div_pi_vec ) > eps_s_bar_div_pi
            Phi_psi_e_node_4(kk, 1) = ( thr_p_plus_1 * pi * V_Phi_Rei_squ_p_plus_1_vec(kk,iiuav) ) ...
                                                            / ( 2 * tanh( ( gamma0 / 2 ) * V_Phi_Rei_div_pi_vec(kk,iiuav) ) );
        else
            Phi_psi_e_node_4(kk, 1) = V_Phi_Rei_div_pi_vec(kk, iiuav) * pi * ...
                                                            ( beta_Phi_1 * ( abs( V_Phi_Rei_div_pi_vec(kk, iiuav) ) ^ 2 ) ...
                                                            + beta_Phi_2 * V_Phi_Rei_squ_2p_vec(kk, iiuav) );
        end
    end
end

== matlab function run_sim_paper_scenario/cal theta_err_ksi agent 4 ==
  data: alfa_theta input; err_ksi_squ_1_node_4 input; theta_err_ksi_1_4 output; err_ksi_squ_2_node_4 input; err_ksi_vec input; theta_err_ksi_2_4 output
function [theta_err_ksi_1_4, theta_err_ksi_2_4] = fcn(alfa_theta, err_ksi_squ_1_node_4, err_ksi_squ_2_node_4, err_ksi_vec)
iiuav = 4;
theta_err_ksi_1_4 = err_ksi_squ_1_node_4(:) .* ( -1 + 2 ./ ( 1 + exp( -alfa_theta .* err_ksi_vec(:,iiuav) ) ) );
theta_err_ksi_2_4 = err_ksi_squ_2_node_4(:) .* ( -1 + 2 ./ ( 1 + exp( -alfa_theta .* err_ksi_vec(:,iiuav) ) ) );

== matlab function run_sim_paper_scenario/cal Phi_psi_e agent 5 ==
  data: Phi_psi_e_node_5 output; beta_Phi_1 input; beta_Phi_2 input; gamma0 input; thr_p_plus_1 input; eps_s_bar_div_pi input; S_bar_vec input; V_Phi_Rei_div_pi_vec input; V_Phi_Rei_squ_p_plus_1_vec input; V_Phi_Rei_squ_2p_vec input
function Phi_psi_e_node_5 = fcn(beta_Phi_1, beta_Phi_2, gamma0, thr_p_plus_1, eps_s_bar_div_pi, ...
                                                            S_bar_vec, V_Phi_Rei_div_pi_vec, ...
                                                            V_Phi_Rei_squ_p_plus_1_vec, V_Phi_Rei_squ_2p_vec)
%%%% intermediate switching rotational error
iiuav = 5;
Phi_psi_e_node_5 = zeros(3,1);
for kk = 1:3
    if S_bar_vec(kk, iiuav) == 0
        Phi_psi_e_node_5(kk, 1) = ( thr_p_plus_1 * pi * V_Phi_Rei_squ_p_plus_1_vec(kk,iiuav) ) ...
                                                        / ( 2 * tanh( ( gamma0 / 2 ) * V_Phi_Rei_div_pi_vec(kk,iiuav) ) );
    else
        if abs( V_Phi_Rei_div_pi_vec ) > eps_s_bar_div_pi
            Phi_psi_e_node_5(kk, 1) = ( thr_p_plus_1 * pi * V_Phi_Rei_squ_p_plus_1_vec(kk,iiuav) ) ...
                                                            / ( 2 * tanh( ( gamma0 / 2 ) * V_Phi_Rei_div_pi_vec(kk,iiuav) ) );
        else
            Phi_psi_e_node_5(kk, 1) = V_Phi_Rei_div_pi_vec(kk, iiuav) * pi * ...
                                                            ( beta_Phi_1 * ( abs( V_Phi_Rei_div_pi_vec(kk, iiuav) ) ^ 2 ) ...
                                                            + beta_Phi_2 * V_Phi_Rei_squ_2p_vec(kk, iiuav) );
        end
    end
end

== matlab function run_sim_paper_scenario/cal Qci agent 1 ==
  data: Qi_vec input; Qci_1 output; Qei_vec input
function Qci_1 = fcn(Qi_vec, Qei_vec)
%%%% quaternion command
iiuav = 1;

sigma1 = Qi_vec(1,iiuav);
q1 = Qi_vec(2:4,iiuav);
sigma2 = Qei_vec(1,iiuav);
q2 = -Qei_vec(2:4,iiuav);

sigma = sigma1*sigma2 - (q1')*q2;
q = sigma1*q2 + sigma2*q1 + cal_askew_mat(q1)*q2;
Qci_1 = [sigma; q];

end

== matlab function run_sim_paper_scenario/cal Qci agent 2 ==
  data: Qi_vec input; Qci_2 output; Qei_vec input
function Qci_2 = fcn(Qi_vec, Qei_vec)
%%%% quaternion command
iiuav = 2;
sigma1 = Qi_vec(1,iiuav);
q1 = Qi_vec(2:4,iiuav);
sigma2 = Qei_vec(1,iiuav);
q2 = -Qei_vec(2:4,iiuav);

sigma = sigma1*sigma2 - (q1')*q2;
q = sigma1*q2 + sigma2*q1 + cal_askew_mat(q1)*q2;
Qci_2 = [sigma; q];

end

== matlab function run_sim_paper_scenario/cal Qci agent 3 ==
  data: Qi_vec input; Qci_3 output; Qei_vec input
function Qci_3 = fcn(Qi_vec, Qei_vec)
%%%% quaternion command
iiuav = 3;
sigma1 = Qi_vec(1,iiuav);
q1 = Qi_vec(2:4,iiuav);
sigma2 = Qei_vec(1,iiuav);
q2 = -Qei_vec(2:4,iiuav);

sigma = sigma1*sigma2 - (q1')*q2;
q = sigma1*q2 + sigma2*q1 + cal_askew_mat(q1)*q2;
Qci_3 = [sigma; q];

end

== matlab function run_sim_paper_scenario/cal Qci agent 4 ==
  data: Qi_vec input; Qci_4 output; Qei_vec input
function Qci_4 = fcn(Qi_vec, Qei_vec)
%%%% quaternion command
iiuav = 4;
sigma1 = Qi_vec(1,iiuav);
q1 = Qi_vec(2:4,iiuav);
sigma2 = Qei_vec(1,iiuav);
q2 = -Qei_vec(2:4,iiuav);

sigma = sigma1*sigma2 - (q1')*q2;
q = sigma1*q2 + sigma2*q1 + cal_askew_mat(q1)*q2;
Qci_4 = [sigma; q];

end

== matlab function run_sim_paper_scenario/cal Qci agent 5 ==
  data: Qi_vec input; Qci_5 output; Qei_vec input
function Qci_5 = fcn(Qi_vec, Qei_vec)
%%%% quaternion command
iiuav = 5;
sigma1 = Qi_vec(1,iiuav);
q1 = Qi_vec(2:4,iiuav);
sigma2 = Qei_vec(1,iiuav);
q2 = -Qei_vec(2:4,iiuav);

sigma = sigma1*sigma2 - (q1')*q2;
q = sigma1*q2 + sigma2*q1 + cal_askew_mat(q1)*q2;
Qci_5 = [sigma; q];

end

== matlab function run_sim_paper_scenario/cal Rci agent 1 ==
  data: Rci_1 output; Qci input
function Rci_1 = fcn(Qci)
%%%% rotation matrix command
thetaci_tmp = Qci(1,1);
qci_tmp = Qci(2:4,1);
Rci_1 = ((thetaci_tmp^2) - (qci_tmp')*qci_tmp) * eye(3,3) ...
                + 2 * qci_tmp * (qci_tmp') ...
                - 2 * thetaci_tmp * cal_askew_mat(qci_tmp);

end

== matlab function run_sim_paper_scenario/cal Rci agent 2 ==
  data: Rci_2 output; Qci input
function Rci_2 = fcn(Qci)
%%%% rotation matrix command

thetaci_tmp = Qci(1,1);
qci_tmp = Qci(2:4,1);
Rci_2 = ((thetaci_tmp^2) - (qci_tmp')*qci_tmp) * eye(3,3) ...
                + 2 * qci_tmp * (qci_tmp') ...
                - 2 * thetaci_tmp * cal_askew_mat(qci_tmp);

end

== matlab function run_sim_paper_scenario/cal Rci agent 3 ==
  data: Rci_3 output; Qci input
function Rci_3 = fcn(Qci)
%%%% rotation matrix command
thetaci_tmp = Qci(1,1);
qci_tmp = Qci(2:4,1);
Rci_3 = ((thetaci_tmp^2) - (qci_tmp')*qci_tmp) * eye(3,3) ...
                + 2 * qci_tmp * (qci_tmp') ...
                - 2 * thetaci_tmp * cal_askew_mat(qci_tmp);

end

== matlab function run_sim_paper_scenario/cal Rci agent 4 ==
  data: Rci_4 output; Qci input
function Rci_4 = fcn(Qci)
%%%% rotation matrix command
thetaci_tmp = Qci(1,1);
qci_tmp = Qci(2:4,1);
Rci_4 = ((thetaci_tmp^2) - (qci_tmp')*qci_tmp) * eye(3,3) ...
                + 2 * qci_tmp * (qci_tmp') ...
                - 2 * thetaci_tmp * cal_askew_mat(qci_tmp);

end

== matlab function run_sim_paper_scenario/cal Rci agent 5 ==
  data: Rci_5 output; Qci_vec input
function Rci_5 = fcn(Qci_vec)
%%%% rotation matrix command
thetaci_tmp = Qci_vec(1,1);
qci_tmp = Qci_vec(2:4,1);
Rci_5 = ((thetaci_tmp^2) - (qci_tmp')*qci_tmp) * eye(3,3) ...
                + 2 * qci_tmp * (qci_tmp') ...
                - 2 * thetaci_tmp * cal_askew_mat(qci_tmp);

end

== matlab function run_sim_paper_scenario/cal Rei agent 1 ==
  data: Rei_1 output; Qei_vec input
function Rei_1 = fcn(Qei_vec)
%%%% rotation matrix error
iiuav = 1;
thetaei_tmp = Qei_vec(1,iiuav);
qei_tmp = Qei_vec(2:4,iiuav);
Rei_1 = ((thetaei_tmp^2) - (qei_tmp')*qei_tmp) * eye(3,3) ...
                + 2 * qei_tmp * (qei_tmp') ...
                - 2 * thetaei_tmp * cal_askew_mat(qei_tmp);

end

== matlab function run_sim_paper_scenario/combine formation control input ==
  data: eta_i_vec output; ksi_i_vec output; eta_1 input; eta_2 input; eta_3 input; eta_4 input; eta_5 input; ksi_1 input; ksi_2 input; ksi_3 input; ksi_4 input; ksi_5 input
function [eta_i_vec, ksi_i_vec] = fcn(eta_1, eta_2, eta_3, eta_4, eta_5, ...
                                                                ksi_1, ksi_2, ksi_3, ksi_4, ksi_5)
eta_i_vec = [eta_1(:), eta_2(:), eta_3(:), eta_4(:), eta_5(:)];
ksi_i_vec = [ksi_1(:), ksi_2(:), ksi_3(:), ksi_4(:), ksi_5(:)];

== matlab function run_sim_paper_scenario/cal Rei agent 2 ==
  data: Rei_2 output; Qei_vec input
function Rei_2 = fcn(Qei_vec)
%%%% rotation matrix error
iiuav = 2;
thetaei_tmp = Qei_vec(1,iiuav);
qei_tmp = Qei_vec(2:4,iiuav);
Rei_2 = ((thetaei_tmp^2) - (qei_tmp')*qei_tmp) * eye(3,3) ...
                + 2 * qei_tmp * (qei_tmp') ...
                - 2 * thetaei_tmp * cal_askew_mat(qei_tmp);

end

== matlab function run_sim_paper_scenario/cal Rei agent 3 ==
  data: Rei_3 output; Qei_vec input
function Rei_3 = fcn(Qei_vec)
%%%% rotation matrix error
iiuav = 3;
thetaei_tmp = Qei_vec(1,iiuav);
qei_tmp = Qei_vec(2:4,iiuav);
Rei_3 = ((thetaei_tmp^2) - (qei_tmp')*qei_tmp) * eye(3,3) ...
                + 2 * qei_tmp * (qei_tmp') ...
                - 2 * thetaei_tmp * cal_askew_mat(qei_tmp);

end

== matlab function run_sim_paper_scenario/cal Rei agent 4 ==
  data: Rei_4 output; Qei_vec input
function Rei_4 = fcn(Qei_vec)
%%%% rotation matrix error
iiuav = 4;
thetaei_tmp = Qei_vec(1,iiuav);
qei_tmp = Qei_vec(2:4,iiuav);
Rei_4 = ((thetaei_tmp^2) - (qei_tmp')*qei_tmp) * eye(3,3) ...
                + 2 * qei_tmp * (qei_tmp') ...
                - 2 * thetaei_tmp * cal_askew_mat(qei_tmp);

end

== matlab function run_sim_paper_scenario/cal Rei agent 5 ==
  data: Rei_5 output; Qei_vec input
function Rei_5 = fcn(Qei_vec)
%%%% rotation matrix error
iiuav = 5;
thetaei_tmp = Qei_vec(1,iiuav);
qei_tmp = Qei_vec(2:4,iiuav);
Rei_5 = ((thetaei_tmp^2) - (qei_tmp')*qei_tmp) * eye(3,3) ...
                + 2 * qei_tmp * (qei_tmp') ...
                - 2 * thetaei_tmp * cal_askew_mat(qei_tmp);

end

== matlab function run_sim_paper_scenario/cal Ri agent 1 ==
  data: Ri_1 output; Qi_vec input
function Ri_1 = fcn(Qi_vec)
%%%% update rotation matrix
iiuav = 1;
thetai_tmp = Qi_vec(1,iiuav);
qi_tmp = Qi_vec(2:4,iiuav);
Ri_1 = ((thetai_tmp^2) - (qi_tmp')*qi_tmp) * eye(3,3) ...
            + 2 * qi_tmp * (qi_tmp') ...
            - 2 * thetai_tmp * cal_askew_mat(qi_tmp);

end

== matlab function run_sim_paper_scenario/cal Ri agent 2 ==
  data: Ri_2 output; Qi_vec input
function Ri_2 = fcn(Qi_vec)
%%%% update rotation matrix
iiuav = 2;
thetai_tmp = Qi_vec(1,iiuav);
qi_tmp = Qi_vec(2:4,iiuav);
Ri_2 = ((thetai_tmp^2) - (qi_tmp')*qi_tmp) * eye(3,3) ...
            + 2 * qi_tmp * (qi_tmp') ...
            - 2 * thetai_tmp * cal_askew_mat(qi_tmp);

end

== matlab function run_sim_paper_scenario/cal Ri agent 3 ==
  data: Ri_3 output; Qi_vec input
function Ri_3 = fcn(Qi_vec)
%%%% update rotation matrix
iiuav = 3;
thetai_tmp = Qi_vec(1,iiuav);
qi_tmp = Qi_vec(2:4,iiuav);
Ri_3 = ((thetai_tmp^2) - (qi_tmp')*qi_tmp) * eye(3,3) ...
            + 2 * qi_tmp * (qi_tmp') ...
            - 2 * thetai_tmp * cal_askew_mat(qi_tmp);

end

== matlab function run_sim_paper_scenario/cal Ri agent 4 ==
  data: Ri_4 output; Qi_vec input
function Ri_4 = fcn(Qi_vec)
%%%% update rotation matrix
iiuav = 4;
thetai_tmp = Qi_vec(1,iiuav);
qi_tmp = Qi_vec(2:4,iiuav);
Ri_4 = ((thetai_tmp^2) - (qi_tmp')*qi_tmp) * eye(3,3) ...
            + 2 * qi_tmp * (qi_tmp') ...
            - 2 * thetai_tmp * cal_askew_mat(qi_tmp);

end

== matlab function run_sim_paper_scenario/cal Ri agent 5 ==
  data: Ri_5 output; Qi_vec input
function Ri_5 = fcn(Qi_vec)
%%%% update rotation matrix
iiuav = 5;
thetai_tmp = Qi_vec(1,iiuav);
qi_tmp = Qi_vec(2:4,iiuav);
Ri_5 = ((thetai_tmp^2) - (qi_tmp')*qi_tmp) * eye(3,3) ...
            + 2 * qi_tmp * (qi_tmp') ...
            - 2 * thetai_tmp * cal_askew_mat(qi_tmp);

end

== matlab function run_sim_paper_scenario/cal S_bar agent 1 ==
  data: cS0 input; gamma0 input; thr_p_plus_1 input; wei_vec input; S_bar_node_1 output; V_Phi_Rei_div_pi_vec input; V_Phi_Rei_squ_p_plus_1_vec input
function S_bar_node_1 = fcn(cS0, gamma0, thr_p_plus_1, wei_vec, ...
                                                        V_Phi_Rei_div_pi_vec, V_Phi_Rei_squ_p_plus_1_vec)
%%%% auxiliary sliding mode surface
iiuav = 1;
S_bar_node_1 = zeros(3,1);
for kk = 1:3
S_bar_node_1(kk,1) = wei_vec(kk,iiuav) + cS0(kk, kk) * ( thr_p_plus_1 * pi * V_Phi_Rei_squ_p_plus_1_vec(kk,iiuav) ) ...
                                        / ( 2 * tanh( ( gamma0 / 2 ) * V_Phi_Rei_div_pi_vec(kk,iiuav) ) );
end

== matlab function run_sim_paper_scenario/cal S_bar agent 2 ==
  data: cS0 input; gamma0 input; thr_p_plus_1 input; wei_vec input; S_bar_node_2 output; V_Phi_Rei_div_pi_vec input; V_Phi_Rei_squ_p_plus_1_vec input
function S_bar_node_2 = fcn(cS0, gamma0, thr_p_plus_1, wei_vec, ...
                                                        V_Phi_Rei_div_pi_vec, V_Phi_Rei_squ_p_plus_1_vec)
%%%% auxiliary sliding mode surface
iiuav = 2;
S_bar_node_2 = zeros(3,1);
for kk = 1:3
S_bar_node_2(kk,1) = wei_vec(kk,iiuav) + cS0(kk, kk) * ( thr_p_plus_1 * pi * V_Phi_Rei_squ_p_plus_1_vec(kk,iiuav) ) ...
                                        / ( 2 * tanh( ( gamma0 / 2 ) * V_Phi_Rei_div_pi_vec(kk,iiuav) ) );
end

== matlab function run_sim_paper_scenario/cal S_bar agent 3 ==
  data: cS0 input; gamma0 input; thr_p_plus_1 input; wei_vec input; S_bar_node_3 output; V_Phi_Rei_div_pi_vec input; V_Phi_Rei_squ_p_plus_1_vec input
function S_bar_node_3 = fcn(cS0, gamma0, thr_p_plus_1, wei_vec, ...
                                                        V_Phi_Rei_div_pi_vec, V_Phi_Rei_squ_p_plus_1_vec)
%%%% auxiliary sliding mode surface
iiuav = 3;
S_bar_node_3 = zeros(3,1);
for kk = 1:3
S_bar_node_3(kk,1) = wei_vec(kk,iiuav) + cS0(kk, kk) * ( thr_p_plus_1 * pi * V_Phi_Rei_squ_p_plus_1_vec(kk,iiuav) ) ...
                                        / ( 2 * tanh( ( gamma0 / 2 ) * V_Phi_Rei_div_pi_vec(kk,iiuav) ) );
end

== matlab function run_sim_paper_scenario/cal S_bar agent 4 ==
  data: cS0 input; gamma0 input; thr_p_plus_1 input; wei_vec input; S_bar_node_4 output; V_Phi_Rei_div_pi_vec input; V_Phi_Rei_squ_p_plus_1_vec input
function S_bar_node_4 = fcn(cS0, gamma0, thr_p_plus_1, wei_vec, ...
                                                        V_Phi_Rei_div_pi_vec, V_Phi_Rei_squ_p_plus_1_vec)
%%%% auxiliary sliding mode surface
iiuav = 4;
S_bar_node_4 = zeros(3,1);
for kk = 1:3
S_bar_node_4(kk,1) = wei_vec(kk,iiuav) + cS0(kk, kk) * ( thr_p_plus_1 * pi * V_Phi_Rei_squ_p_plus_1_vec(kk,iiuav) ) ...
                                        / ( 2 * tanh( ( gamma0 / 2 ) * V_Phi_Rei_div_pi_vec(kk,iiuav) ) );
end

== matlab function run_sim_paper_scenario/cal S_bar agent 5 ==
  data: cS0 input; gamma0 input; thr_p_plus_1 input; wei_vec input; S_bar_node_5 output; V_Phi_Rei_div_pi_vec input; V_Phi_Rei_squ_p_plus_1_vec input
function S_bar_node_5 = fcn(cS0, gamma0, thr_p_plus_1, wei_vec, ...
                                                        V_Phi_Rei_div_pi_vec, V_Phi_Rei_squ_p_plus_1_vec)
%%%% auxiliary sliding mode surface
iiuav = 5;
S_bar_node_5 = zeros(3,1);
for kk = 1:3
S_bar_node_5(kk,1) = wei_vec(kk,iiuav) + cS0(kk, kk) * ( thr_p_plus_1 * pi * V_Phi_Rei_squ_p_plus_1_vec(kk,iiuav) ) ...
                                        / ( 2 * tanh( ( gamma0 / 2 ) * V_Phi_Rei_div_pi_vec(kk,iiuav) ) );
end

== matlab function run_sim_paper_scenario/cal Si agent 1 ==
  data: cS0 input; wei_vec input; Phi_psi_e_vec input; Si_1 output
function Si_1 = fcn(cS0, wei_vec, Phi_psi_e_vec)
%%%% sliding mode surface
iiuav = 1;
Si_1 = zeros(3,1);
for kk = 1:3
    Si_1(kk, 1) = wei_vec(kk, iiuav) + cS0(kk, kk) * Phi_psi_e_vec(kk, iiuav);
end

== matlab function run_sim_paper_scenario/cal Si agent 2 ==
  data: cS0 input; wei_vec input; Phi_psi_e_vec input; Si_2 output
function Si_2 = fcn(cS0, wei_vec, Phi_psi_e_vec)
%%%% sliding mode surface
iiuav = 2;
Si_2 = zeros(3,1);
for kk = 1:3
    Si_2(kk, 1) = wei_vec(kk, iiuav) + cS0(kk, kk) * Phi_psi_e_vec(kk, iiuav);
end

== matlab function run_sim_paper_scenario/cal Si agent 3 ==
  data: cS0 input; wei_vec input; Phi_psi_e_vec input; Si_3 output
function Si_3 = fcn(cS0, wei_vec, Phi_psi_e_vec)
%%%% sliding mode surface
iiuav = 3;
Si_3 = zeros(3,1);
for kk = 1:3
    Si_3(kk, 1) = wei_vec(kk, iiuav) + cS0(kk, kk) * Phi_psi_e_vec(kk, iiuav);
end

== matlab function run_sim_paper_scenario/cal Si agent 4 ==
  data: cS0 input; wei_vec input; Phi_psi_e_vec input; Si_4 output
function Si_4 = fcn(cS0, wei_vec, Phi_psi_e_vec)
%%%% sliding mode surface
iiuav = 4;
Si_4 = zeros(3,1);
for kk = 1:3
    Si_4(kk, 1) = wei_vec(kk, iiuav) + cS0(kk, kk) * Phi_psi_e_vec(kk, iiuav);
end

== matlab function run_sim_paper_scenario/cal Si agent 5 ==
  data: cS0 input; wei_vec input; Phi_psi_e_vec input; Si_5 output
function Si_5 = fcn(cS0, wei_vec, Phi_psi_e_vec)
%%%% sliding mode surface
iiuav = 5;
Si_5 = zeros(3,1);
for kk = 1:3
    Si_5(kk, 1) = wei_vec(kk, iiuav) + cS0(kk, kk) * Phi_psi_e_vec(kk, iiuav);
end

== matlab function run_sim_paper_scenario/cal abs 61 ==
  data: x input; y output
function y = fcn(x)
y = abs(x(:));

== matlab function run_sim_paper_scenario/choose ksi_est_err 7 ==
  data: x input; y output
function y = fcn(x)
iiuav = 4;
y = x(:,iiuav);

== matlab function run_sim_paper_scenario/cal abs 62 ==
  data: x input; y output
function y = fcn(x)
y = abs(x(:));

== matlab function run_sim_paper_scenario/cal abs 63 ==
  data: x input; y output
function y = fcn(x)
y = abs(x(:));

== matlab function run_sim_paper_scenario/cal abs 64 ==
  data: x input; y output
function y = fcn(x)
y = abs(x(:));

== matlab function run_sim_paper_scenario/cal abs 65 ==
  data: x input; y output
function y = fcn(x)
y = abs(x(:));

== matlab function run_sim_paper_scenario/cal abs 66 ==
  data: x input; y output
function y = fcn(x)
y = abs(x(:));

== matlab function run_sim_paper_scenario/cal abs 67 ==
  data: x input; y output
function y = fcn(x)
y = abs(x(:));

== matlab function run_sim_paper_scenario/cal abs 68 ==
  data: x input; y output
function y = fcn(x)
y = abs(x(:));

== matlab function run_sim_paper_scenario/cal abs 69 ==
  data: x input; y output
function y = fcn(x)
y = abs(x(:));

== matlab function run_sim_paper_scenario/cal abs 70 ==
  data: x input; y output
function y = fcn(x)
y = abs(x(:));

== matlab function run_sim_paper_scenario/cal abs 71 ==
  data: x input; y output
function y = fcn(x)
y = abs(x(:));

== matlab function run_sim_paper_scenario/choose ksi_est_err 8 ==
  data: x input; y output
function y = fcn(x)
iiuav = 4;
y = x(:,iiuav);
